simulink model "traj_gene_normal"  (R2018b)
settings: Solver=ode4  StartTime=0.0  StopTime=T  FixedStep=dt_solve  RelTol=1e-3
InitFcn:
  | traj_init_normal;
values from neighbouring files (symbols this model uses):
  f_harmful = cross(2*wien+wenn,v)    [traj_init_normal.m]
undefined symbols (not defined in the file or in its folder): Earth, WGS84
libraries: aerolibgravity2 x2, aerolibutil x2, sharedtransform x2, aerolib6dof2 x1
settings Model: ModifiedComment=longt -- Mon Nov 05 19:40:50 2018 -- Version 1.9  Creator=longteng  LastModifiedBy=longt
settings DataIOCC: SaveOutput=off  SignalLogging=off  DSMLogging=off  SaveTime=off
settings DebuggingCC: LibraryContextMissingDiagnostic=none
settings SFSimCC: SimUseLocalCustomCode=off
settings RTWCC: RTWUseLocalCustomCode=off

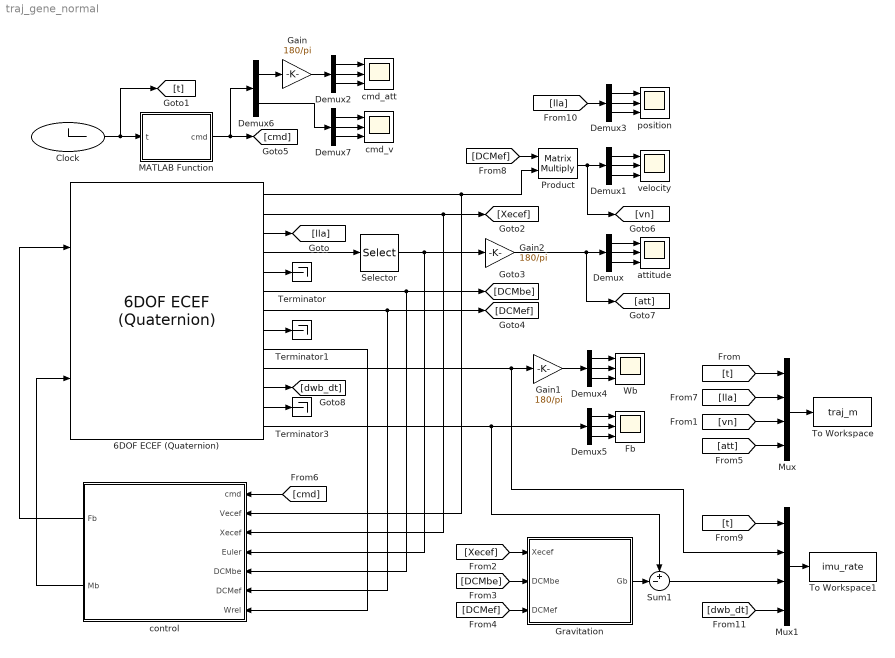
== system traj_gene_normal ==
  6DOF ECEF (Quaternion) : aerolib6dof2/6DOF ECEF (Quaternion)  units=Metric (MKS)  mtype=Fixed  xg_0=p0  Vm_0=vb0  eul_0=att0  pm_0=[0 0 0]  mass_0=1.0  mass_e=0.5  mass_f=2.0  inertia=eye(3)  inertia_e=eye(3)  inertia_f=2*eye(3)  vre_flag=on  abi_flag=on  ptype=Earth (WGS84)  R=6378137  F=1/298.257223563  w_E=7292115e-11  angle_in=Internal  LG0=0  quat_statename=''  pm_statename=''  Vm_statename=''  posECEF_statename=''  posECI_statename=''  LG_statename=''  mass_statename=''
      settings: SourceProductName=Aerospace Blockset  SourceProductBaseCode=AE
  Clock : Clock
  Demux{,1..5,7} (7 alike) : Demux  Outputs=3
  Demux6 : Demux  Outputs=[3 3]
  Fb : Scope  NumInputPorts=3
  Gain : Gain  Gain=180/pi
  Gain1 : Gain  Gain=180/pi
  Gain2 : Gain  Gain=180/pi
  Gravitation : Subsystem
  MATLAB Function : MATLAB Function  TreatAsAtomicUnit=on
  Mux : Mux
  Mux1 : Mux
  Product : Product  Multiplication=Matrix(*)
  Selector : Selector  InputPortWidth=3  IndexOptions=Index vector (dialog)  Indices=[3 2 1]  OutputSizes=1
  Sum1 : Sum  Inputs=+-|
  Terminator : Terminator
  Terminator1 : Terminator
  Terminator3 : Terminator
  To Workspace : ToWorkspace  VariableName=traj_m  SampleTime=-1
      settings: Decimation=dt_traj/dt_solve
  To Workspace1 : ToWorkspace  VariableName=imu_rate  SampleTime=-1
      settings: Decimation=dt_imu_rate/dt_solve
  Wb : Scope  NumInputPorts=3
  attitude : Scope  NumInputPorts=3
  cmd_att : Scope  NumInputPorts=3
  cmd_v : Scope  NumInputPorts=3
  control : Subsystem
  position : Scope  NumInputPorts=3
  velocity : Scope  NumInputPorts=3
  wires:
  Demux/1 -> attitude/1
  Demux/2 -> attitude/2
  Demux/3 -> attitude/3
  Demux3/1 -> position/1
  Demux3/2 -> position/2
  Demux3/3 -> position/3
  6DOF ECEF (Quaternion)/1 -> Product/2, control/2(Vecef)
  6DOF ECEF (Quaternion)/2 -> [Xecef], control/3(Xecef)
  6DOF ECEF (Quaternion)/4 -> Selector/1
  6DOF ECEF (Quaternion)/6 -> [DCMbe], control/5(DCMbe)
  6DOF ECEF (Quaternion)/7 -> [DCMef], control/6(DCMef)
  control/1(Fb) -> 6DOF ECEF (Quaternion)/1
  Demux1/3 -> velocity/3
  Demux1/2 -> velocity/2
  Demux1/1 -> velocity/1
  control/2(Mb) -> 6DOF ECEF (Quaternion)/2
  6DOF ECEF (Quaternion)/9 -> control/7(Wrel)
  Gain2/1 -> [att], Demux/1
  Product/1 -> [vn], Demux1/1
  Demux4/1 -> Wb/1
  Demux4/2 -> Wb/2
  Demux4/3 -> Wb/3
  Demux5/1 -> Fb/1
  Demux5/2 -> Fb/2
  Demux5/3 -> Fb/3
  6DOF ECEF (Quaternion)/5 -> Terminator/1
  6DOF ECEF (Quaternion)/8 -> Terminator1/1
  6DOF ECEF (Quaternion)/12 -> Terminator3/1
  Mux/1 -> To Workspace/1
  [DCMbe] -> Gravitation/2(DCMbe)
  [Xecef] -> Gravitation/1(Xecef)
  [DCMef] -> Gravitation/3(DCMef)
  Gravitation/1(Gb) -> Sum1/2
  6DOF ECEF (Quaternion)/11 -> [dwb_dt]
  6DOF ECEF (Quaternion)/13 -> Demux5/1, Sum1/1
  [DCMef] -> Product/1
  Mux1/1 -> To Workspace1/1
  Selector/1 -> Gain2/1, control/4(Euler)
  Clock/1 -> [t], MATLAB Function/1(t)
  MATLAB Function/1(cmd) -> Demux6/1, [cmd]
  [t] -> Mux/1
  [lla] -> Mux/2
  [vn] -> Mux/3
  [att] -> Mux/4
  [cmd] -> control/1(cmd)
  Gain1/1 -> Demux4/1
  6DOF ECEF (Quaternion)/10 -> Gain1/1, Mux1/2
  Sum1/1 -> Mux1/3
  [t] -> Mux1/1
  Demux2/3 -> cmd_att/3
  Demux2/2 -> cmd_att/2
  Demux2/1 -> cmd_att/1
  Demux7/1 -> cmd_v/1
  Demux7/2 -> cmd_v/2
  Demux7/3 -> cmd_v/3
  Demux6/1 -> Gain/1
  Demux6/2 -> Demux7/1
  6DOF ECEF (Quaternion)/3 -> [lla]
  [lla] -> Demux3/1
  Gain/1 -> Demux2/1
  [dwb_dt] -> Mux1/4

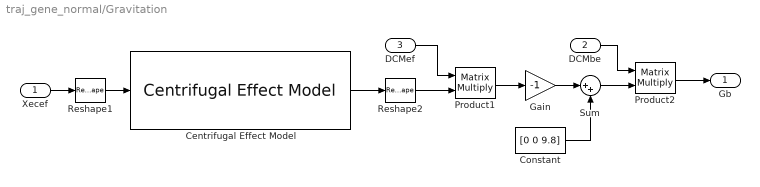
== system traj_gene_normal/Gravitation ==
  Xecef : Inport
  DCMbe : Inport  Port=2
  DCMef : Inport  Port=3
  Centrifugal Effect Model : aerolibgravity2/Centrifugal Effect Model  ptype=Earth  omega=7.2921150e-05  rate_loc=off
      settings: SourceProductName=Aerospace Blockset  SourceProductBaseCode=AE
  Constant : Constant  Value=[0 0 9.8]
  Gain : Gain  Gain=-1
  Product1 : Product  Multiplication=Matrix(*)
  Product2 : Product  Multiplication=Matrix(*)
  Reshape1 : Reshape
  Reshape2 : Reshape
  Sum : Sum  Inputs=|++
  Gb : Outport
  wires:
  Product2/1 -> Gb/1
  Reshape1/1 -> Centrifugal Effect Model/1
  Reshape2/1 -> Product1/2
  Centrifugal Effect Model/1 -> Reshape2/1
  DCMbe/1 -> Product2/1
  Xecef/1 -> Reshape1/1
  DCMef/1 -> Product1/1
  Product1/1 -> Gain/1
  Sum/1 -> Product2/2
  Gain/1 -> Sum/1
  Constant/1 -> Sum/2

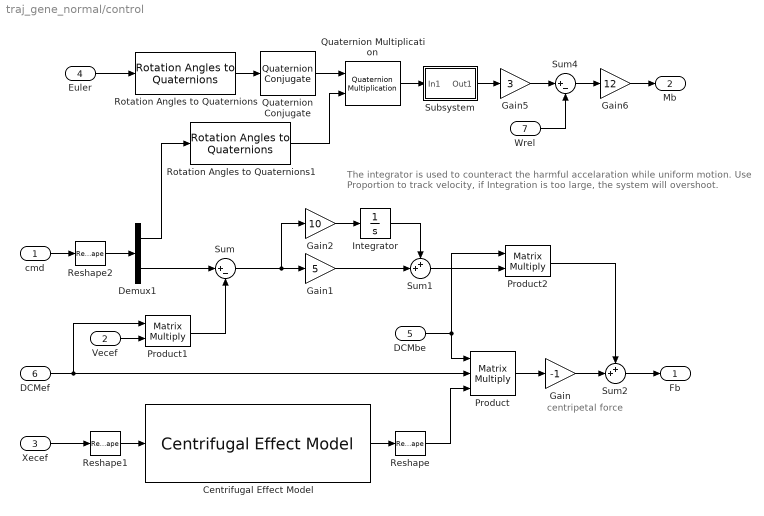
== system traj_gene_normal/control ==
  note: The integrator is used to counteract the harmful accelaration while uniform motion.
      | Use Proportion to track velocity, if Integration is too large, the system will overshoot.
  note: centripetal force
  cmd : Inport
  Vecef : Inport  Port=2
  Xecef : Inport  Port=3
  Euler : Inport  Port=4
  DCMbe : Inport  Port=5
  DCMef : Inport  Port=6
  Wrel : Inport  Port=7
  Centrifugal Effect Model : aerolibgravity2/Centrifugal Effect Model  ptype=Earth  omega=7.2921150e-05  rate_loc=off
      settings: SourceProductName=Aerospace Blockset  SourceProductBaseCode=AE
  Demux1 : Demux  Outputs=[3 3]
  Gain : Gain  Gain=-1
  Gain1 : Gain  Gain=5
  Gain2 : Gain  Gain=10
  Gain5 : Gain  Gain=3
  Gain6 : Gain  Gain=12
  Integrator : Integrator  InitialCondition=f_harmful  LimitOutput=on  UpperSaturationLimit=0.2  LowerSaturationLimit=-0.2
  Product : Product  Inputs=3  Multiplication=Matrix(*)
  Product1 : Product  Multiplication=Matrix(*)
  Product2 : Product  Multiplication=Matrix(*)
  Quaternion Conjugate : aerolibutil/Quaternion Conjugate
      settings: SourceProductName=Aerospace Blockset  SourceProductBaseCode=AE
  Quaternion Multiplication : aerolibutil/Quaternion Multiplication
  Reshape : Reshape
  Reshape1 : Reshape
  Reshape2 : Reshape
  Rotation Angles to Quaternions : sharedtransform/Rotation Angles to Quaternions  rotationOrder=ZYX  aMode=aMode
      settings: SourceProductName=Aerospace Blockset  SourceProductBaseCode=AE
  Rotation Angles to Quaternions1 : sharedtransform/Rotation Angles to Quaternions  rotationOrder=ZYX  aMode=aMode
      settings: SourceProductName=Aerospace Blockset  SourceProductBaseCode=AE
  Subsystem : Subsystem
  Sum : Sum  Inputs=|+-
  Sum1 : Sum  Inputs=++|
  Sum2 : Sum  Inputs=++|
  Sum4 : Sum  Inputs=|+-
  Fb : Outport
  Mb : Outport  Port=2
  wires:
  Sum2/1 -> Fb/1
  Product1/1 -> Sum/2
  Gain2/1 -> Integrator/1
  Product2/1 -> Sum2/1
  Gain/1 -> Sum2/2
  Vecef/1 -> Product1/2
  Centrifugal Effect Model/1 -> Reshape/1
  DCMbe/1 -> Product/1, Product2/1
  Reshape/1 -> Product/3
  cmd/1 -> Reshape2/1
  Integrator/1 -> Sum1/1
  Gain1/1 -> Sum1/2
  Xecef/1 -> Reshape1/1
  Product/1 -> Gain/1
  DCMef/1 -> Product1/1, Product/2
  Reshape1/1 -> Centrifugal Effect Model/1
  Wrel/1 -> Sum4/2
  Sum4/1 -> Gain6/1
  Gain6/1 -> Mb/1
  Sum1/1 -> Product2/2
  Euler/1 -> Rotation Angles to Quaternions/1
  Rotation Angles to Quaternions/1 -> Quaternion Conjugate/1
  Rotation Angles to Quaternions1/1 -> Quaternion Multiplication/2
  Quaternion Conjugate/1 -> Quaternion Multiplication/1
  Gain5/1 -> Sum4/1
  Quaternion Multiplication/1 -> Subsystem/1(In1)
  Subsystem/1(Out1) -> Gain5/1
  Sum/1 -> Gain2/1, Gain1/1
  Demux1/2 -> Sum/1
  Demux1/1 -> Rotation Angles to Quaternions1/1
  Reshape2/1 -> Demux1/1

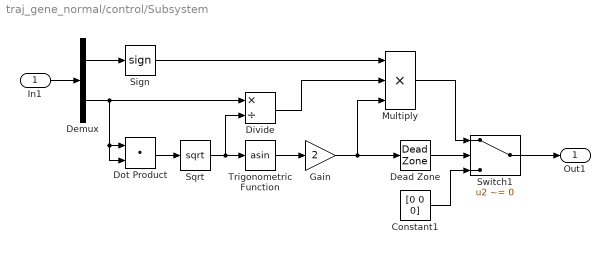
== system traj_gene_normal/control/Subsystem ==
  In1 : Inport
  Constant1 : Constant  Value=[0 0 0]
  Dead Zone : DeadZone  LowerValue=-1e-12  UpperValue=1e-12  SaturateOnIntegerOverflow=on
  Demux : Demux  Outputs=[1 3]
  Divide : Product  Inputs=*/
  Dot Product : DotProduct  InputSameDT=on  OutDataTypeStr=Inherit: Inherit via internal rule
  Gain : Gain  Gain=2
  Multiply : Product  Inputs=3
  Sign : Signum
  Sqrt : Sqrt  SaturateOnIntegerOverflow=on
  Switch1 : Switch  Criteria=u2 ~= 0
  Trigonometric Function : Trigonometry  Operator=asin
  Out1 : Outport
  wires:
  In1/1 -> Demux/1
  Trigonometric Function/1 -> Gain/1
  Constant1/1 -> Switch1/3
  Switch1/1 -> Out1/1
  Multiply/1 -> Switch1/1
  Sqrt/1 -> Trigonometric Function/1, Divide/2
  Dot Product/1 -> Sqrt/1
  Demux/2 -> Dot Product/2, Dot Product/1, Divide/1
  Demux/1 -> Sign/1
  Divide/1 -> Multiply/2
  Gain/1 -> Dead Zone/1, Multiply/3
  Sign/1 -> Multiply/1
  Dead Zone/1 -> Switch1/2

== matlab function traj_gene_normal/MATLAB Function ==
  data: t input; cmd output
function cmd = fcn(t)

cmd = traj_design(t);

end
